simulink model "lab_3simulink"  (R2023a)
settings: Solver=VariableStepAuto  StartTime=0.0  StopTime=10.0  RelTol=1e-3
settings Model: Creator=george theologis  LastModifiedBy=george theologis

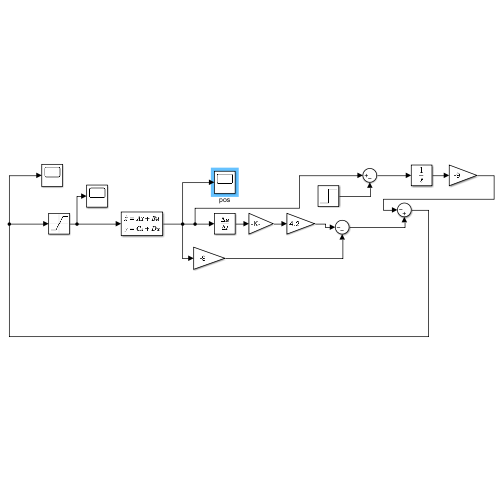
[thumbnail: Simulink's stored preview of the top-level diagram]
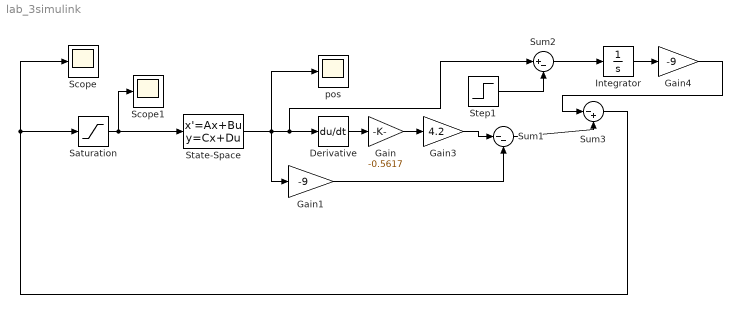
== system lab_3simulink ==
  Derivative : Derivative
  Gain : Gain  Gain=-0.5617
  Gain1 : Gain  Gain=-9
  Gain3 : Gain  Gain=4.2
  Gain4 : Gain  Gain=-9
  Integrator : Integrator
  Saturation : Saturate  UpperLimit=10  LowerLimit=-10
  Scope : Scope
  Scope1 : Scope
  State-Space : StateSpace  A=|  B=[0;1.6906;]  C=[1 0]  D=0  InitialCondition=[2;0;]
      | [0 -1.7802
      | ;0 -1/0.53;]
  Step1 : Step  Time=0  After=5  SampleTime=0
  Sum1 : Sum  Inputs=|--
  Sum2 : Sum  Inputs=|+-
  Sum3 : Sum  Inputs=|-+
  pos : Scope
  wires:
  Gain3/1 -> Sum1/1
  Saturation/1 -> State-Space/1, Scope1/1
  Gain1/1 -> Sum1/2
  Gain/1 -> Gain3/1
  Derivative/1 -> Gain/1
  State-Space/1 -> Sum2/1, Derivative/1, Gain1/1, pos/1
  Step1/1 -> Sum2/2
  Sum2/1 -> Integrator/1
  Sum3/1 -> Scope/1, Saturation/1
  Integrator/1 -> Gain4/1
  Gain4/1 -> Sum3/1
  Sum1/1 -> Sum3/2
